simulink model "BPRZ_AMI_and_AMI"  (R2018a)
settings: Solver=VariableStepAuto  StartTime=0.0  StopTime=50  RelTol=1e-3
libraries: commrandsrc3 x1, simulink_extras x1, commutil2 x1
settings Model: Creator=Souhardhya Paul  LastModifiedBy=Souhardhya Paul

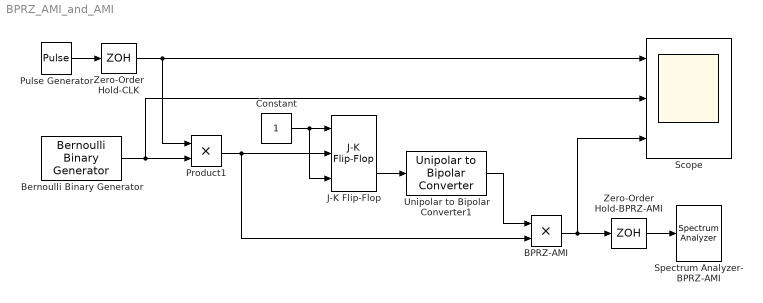
== system BPRZ_AMI_and_AMI ==
  BPRZ-AMI : Product
  Bernoulli Binary Generator : commrandsrc3/Bernoulli Binary Generator  ProbabilityOfZero=0.5  SeedSource=Auto  Seed=0  SampleTime=0.1  SamplesPerFrame=1  OutputDataType=boolean  SimulateUsing=Interpreted execution
  Constant : Constant  OutDataTypeStr=boolean
  J-K Flip-Flop : simulink_extras/Flip Flops/J-K Flip-Flop  initial_condition=0
      settings: SourceProductName=Simulink
  Product1 : Product
  Pulse Generator : DiscretePulseGenerator  PulseType=Time based  Period=0.1  PulseWidth=50  SampleTime=0.1
  Scope : Scope  NumInputPorts=3
  Spectrum Analyzer- BPRZ-AMI : SpectrumAnalyzer
  Unipolar to Bipolar Converter1 : commutil2/Unipolar to Bipolar Converter  M=2  polarity=Positive  dataType=Inherit via internal rule
      settings: SourceProductName=Communications System Toolbox
  Zero-Order Hold-BPRZ-AMI : ZeroOrderHold  SampleTime=0.01
  Zero-Order Hold-CLK : ZeroOrderHold  SampleTime=0.05
  wires:
  Bernoulli Binary Generator/1 -> Scope/2, Product1/2
  Zero-Order Hold-CLK/1 -> Product1/1, Scope/1
  Product1/1 -> BPRZ-AMI/2, J-K Flip-Flop/2
  Unipolar to Bipolar Converter1/1 -> BPRZ-AMI/1
  BPRZ-AMI/1 -> Zero-Order Hold-BPRZ-AMI/1, Scope/3
  J-K Flip-Flop/2 -> Unipolar to Bipolar Converter1/1
  Constant/1 -> J-K Flip-Flop/3, J-K Flip-Flop/1
  Zero-Order Hold-BPRZ-AMI/1 -> Spectrum Analyzer- BPRZ-AMI/1
  Pulse Generator/1 -> Zero-Order Hold-CLK/1
